simulink model "sf_elevator"  (R2017b)
settings: Solver=FixedStepDiscrete  StartTime=0.0  StopTime=inf  FixedStep=0.01  RelTol=1e-3  EnableMultiTasking=on
InitFcn:
  | allCarIds = [1 2];
StartFcn:
  | root = sfroot;
  | data = root.find('-isa','Stateflow.Data');
  | posA = data.find('Name','A_position').Props.InitialValue;
  | posB = data.find('Name','B_position').Props.InitialValue;
  | sf_elevator_gui('init', 'sf_elevator', allCarIds, [posA posB]);
StopFcn:
  | sf_elevator_gui('close');
undefined symbols (not defined in the file): Stateflow
libraries: sf_elevator_lib x2, sf_gui_elevator_controller_lib x2
CloseFcn:
  | sf_elevator_gui('close');
  | clear allCarIds;
settings Model: ExtModeAutoUpdateStatusClock=off  Creator=The MathWorks, Inc.  LastModifiedBy=The MathWorks, Inc.
settings DataIOCC: LimitDataPoints=on  SaveFormat=StructureWithTime  SignalLoggingName=sigsOut
settings OptimizationCC: ExpressionDepthLimit=2147483647  InitFltsAndDblsToZero=on  EfficientMapNaN2IntZero=off  LifeSpan=Inf
settings DebuggingCC: SaveWithParameterizedLinksMsg=none  UnderspecifiedInitializationDetection=Classic  MergeDetectMultiDrivingBlocksExec=none  SignalResolutionControl=TryResolveAllWithWarning  MultiTaskDSMMsg=warning  MultiTaskCondExecSysMsg=none  FcnCallInpInsideContextMsg=warning  AllowSymbolicDim=off  StateNameClashWarn=warning  SFUnexpectedBacktrackingDiag=warning  SFNoUnconditionalDefaultTransitionDiag=warning  SFExecutionAtInitializationDiag=none
settings HardwareCC: ProdBitPerPointer=32  ProdBitPerSizeT=32  ProdBitPerPtrDiffT=32  ProdLargestAtomicFloat=None  ProdIntDivRoundTo=Undefined  ProdEndianess=Unspecified  ProdWordSize=32  ProdHWDeviceType=32-bit Generic  TargetBitPerLong=64  TargetBitPerPointer=64  TargetBitPerSizeT=64  TargetBitPerPtrDiffT=64  TargetLongLongMode=on  TargetIntDivRoundTo=Zero  TargetEndianess=LittleEndian  TargetWordSize=64  TargetHWDeviceType=MATLAB Host  ProdEqTarget=off
settings ModelReferenceCC: PropagateSignalLabelsOutOfModel=off
settings SFSimCC: SFSimEcho=off  SimIntegrity=off  SimParseCustomCode=off
settings RTWCC: SystemTargetFile=ert.tlc  TemplateMakefile=ert_default_tmf  Description=Real-Time Workshop Embedded Coder  GenerateReport=on  IncludeHyperlinkInReport=on  LaunchReport=on  GenerateTraceInfo=on  GenerateTraceReport=on  GenerateTraceReportSl=on  GenerateTraceReportSf=on  GenerateTraceReportEml=on
settings CodeAppCC: IgnoreCustomStorageClasses=off  CustomSymbolStrType=$N$R$M  CustomSymbolStrModelFcn=$N  StateflowObjectComments=on  InternalIdentifier=Classic
settings ERTTargetCC: MultiwordLength=2048  GenerateSampleERTMain=on  ERTCustomFileTemplate=example_file_process.tlc  ConvertIfToSwitch=off  SuppressUnreachableDefaultCases=off
settings ConfigComp: CovMetricSettings=dcmtr  CovHtmlReporting=on  CovSaveCumulativeToWorkspaceVar=on  CovSaveSingleToWorkspaceVar=on  CovExternalEMLEnable=off  CovSFcnEnable=off

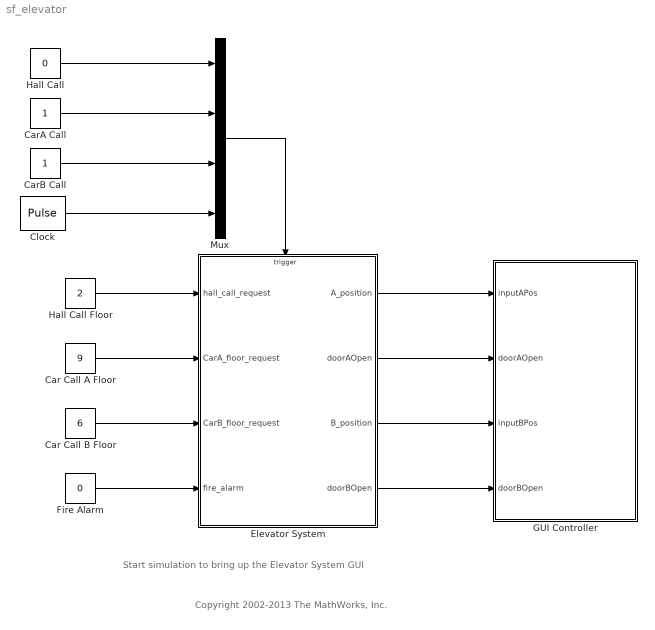
== system sf_elevator ==
  note: Start simulation to bring up the Elevator System GUI
  note: Copyright 2002-2013 The MathWorks, Inc.
  Car Call A Floor : Constant  Value=9  OutDataTypeStr=uint8
  Car Call B Floor : Constant  Value=6  OutDataTypeStr=uint8
  CarA Call : Constant  OutDataTypeStr=double
  CarB Call : Constant  OutDataTypeStr=double
  Clock : DiscretePulseGenerator  PulseType=Time based  PulseWidth=50
  Elevator System : Stateflow chart  TreatAsAtomicUnit=on
  Fire Alarm : Constant  Value=0  OutDataTypeStr=boolean
  GUI Controller : Stateflow chart  TreatAsAtomicUnit=on
  Hall Call : Constant  Value=0  OutDataTypeStr=double
  Hall Call Floor : Constant  Value=2  OutDataTypeStr=uint8
  Mux : Mux
  wires:
  Elevator System/1(A_position) -> GUI Controller/1(inputAPos)
  Elevator System/2(doorAOpen) -> GUI Controller/2(doorAOpen)
  Elevator System/3(B_position) -> GUI Controller/3(inputBPos)
  Elevator System/4(doorBOpen) -> GUI Controller/4(doorBOpen)
  Hall Call/1 -> Mux/1
  CarA Call/1 -> Mux/2
  CarB Call/1 -> Mux/3
  Clock/1 -> Mux/4
  Mux/1 -> Elevator System/Trigger
  Hall Call Floor/1 -> Elevator System/1(hall_call_request)
  Car Call A Floor/1 -> Elevator System/2(CarA_floor_request)
  Car Call B Floor/1 -> Elevator System/3(CarB_floor_request)
  Fire Alarm/1 -> Elevator System/4(fire_alarm)

== stateflow chart sf_elevator/Elevator System ==
  state Elevator_Manager [parallel]
    settings: executionOrder=1
    state register(hall_call_floor) [function]
      (default) -> (junction 2062) : {enqueue(hall_call_floor);
          | hall_call_status[hall_call_floor] = 1;}
    state enqueue(hall_call_floor) [function]
      (default) -> (junction 1513)
      (junction 1513) -> (junction 1514) [order 1] : [hall_call_status[hall_call_floor] != 0]
      (junction 1513) -> (junction 1516) [order 2] : {i = 0;}
      (junction 1516) -> (junction 1515) [order 1] : [hall_call_queue[i] == hall_call_floor]
      (junction 1516) -> (junction 1516) [order 2] : [hall_call_queue[i] > 0 && i<NUM_FLOOR]{i++;}
      (junction 1516) -> (junction 1517) [order 3]
      (junction 1517) -> (junction 1518) [order 1] : [i >= NUM_FLOOR]
      (junction 1517) -> (junction 1519) [order 2] : {hall_call_queue[i] = hall_call_floor;}
    state process_hall_call [function]
      (default) -> (junction 2070)
      (junction 2070) -> (junction 2072) : {
          | /* 'INIT':Initialization */
          | request_floor = hall_call_queue[0];
          | }
      (junction 2072) -> (junction 2074) : {
          | /* Fire alarm is on */
          | fire_alarm_on = (fire_alarm);
          | }
      (junction 2074) -> (junction 2076) : {
          | /* There is outstanding request */
          | request_outstanding = (request_floor > 0);
          | }
      (junction 2076) -> (junction 2078) : {
          | /* Elevator A is idle */
          | elevator_A_idle = (Elevator_A.get_status() == ElevatorStatus.IDLE);
          | }
      (junction 2078) -> (junction 2080) : {
          | /* Elevator B is idle */
          | elevator_B_idle = (Elevator_B.get_status() == ElevatorStatus.IDLE);
          | }
      (junction 2080) -> (junction 2082) : {
          | /* Elevator A is closer to request */
          | elevator_A_closer = (fabs(Elevator_A.get_position() - request_floor) <= fabs(Elevator_B.get_position() - request_floor));
          | }
      (junction 2082) -> (junction 2084) [order 1] : [fire_alarm_on]
      (junction 2084) -> (junction 2086) : {
          | /* 'EMR':Emergency */
          | Elevator_A.register(floor(Elevator_A.get_position()+Elevator_A.get_direction()/2));
          | Elevator_B.register(floor(Elevator_B.get_position()+Elevator_B.get_direction()/2));
          | }
      (junction 2082) -> (junction 2088) [order 2]
      (junction 2088) -> (junction 2090) [order 1] : [!request_outstanding]
      (junction 2090) -> (junction 2092) : {
          | /* 'NONE':Both elevators are busy, OR no request present */
          |
          | }
      (junction 2088) -> (junction 2094) [order 2]
      (junction 2094) -> (junction 2096) [order 1] : [!elevator_A_idle && !elevator_B_idle]
      (junction 2096) -> (junction 2098) : {
          | /* 'NONE':Both elevators are busy, OR no request present */
          |
          | }
      (junction 2094) -> (junction 2100) [order 2]
      (junction 2100) -> (junction 2102) [order 1] : [elevator_A_idle && !elevator_B_idle]
      (junction 2102) -> (junction 2104) : {
          | /* 'A':Elevator A should respond to request */
          | Elevator_A.enqueue(request_floor);
          | Main_dequeue(request_floor);
          | }
      (junction 2100) -> (junction 2106) [order 2]
      (junction 2106) -> (junction 2108) [order 1] : [!elevator_A_idle && elevator_B_idle]
      (junction 2108) -> (junction 2110) : {
          | /* 'B':Elevator B should respond to request */
          | Elevator_B.enqueue(request_floor);
          | Main_dequeue(request_floor);
          | }
      (junction 2106) -> (junction 2112) [order 2]
      (junction 2112) -> (junction 2114) [order 1] : [elevator_A_idle && elevator_B_idle && elevator_A_closer]
      (junction 2114) -> (junction 2116) : {
          | /* 'A':Elevator A should respond to request */
          | Elevator_A.enqueue(request_floor);
          | Main_dequeue(request_floor);
          | }
      (junction 2112) -> (junction 2118) [order 2]
      (junction 2118) -> (junction 2120) [order 1] : [elevator_A_idle && elevator_B_idle && !elevator_A_closer]
      (junction 2120) -> (junction 2122) : {
          | /* 'B':Elevator B should respond to request */
          | Elevator_B.enqueue(request_floor);
          | Main_dequeue(request_floor);
          | }
      (junction 2118) -> (junction 2124) [order 2]
    Elevator_Manager -> (junction 2054) [order 1] : HALL_CALL {register(hall_call_request);}
    Elevator_Manager -> (junction 2057) [order 2] : CLOCK {process_hall_call();} //Clock drives whole system
  state result = Main_exists_in_queue(floor) [function]
    (default) -> (junction 1904) : {i=0;}
    (junction 1904) -> (junction 1904) [order 1] : [hall_call_queue[i] > 0 && ...
        | i<NUM_FLOOR && ...
        | hall_call_queue[i] != floor]{i++;}
    (junction 1904) -> (junction 1905) [order 2]
    (junction 1905) -> (junction 1906) [order 1] : [i >= NUM_FLOOR || hall_call_queue[i] == 0]{result = 0;}
    (junction 1905) -> (junction 1907) [order 2] : {result = i+1;}
  state Main_deregister(hall_call_floor) [function]
    (default) -> (junction 1898) : {Main_dequeue(hall_call_floor);
        | hall_call_status[hall_call_floor] = 0;}
  state Elevator_A [parallel]
    settings: executionOrder=2
  state Main_dequeue(hall_call_floor) [function]
    (default) -> (junction 1916) : {i=0;}
    (junction 1916) -> (junction 1916) [order 1] : [hall_call_queue[i] > 0 && ...
        | i<NUM_FLOOR && ...
        | hall_call_queue[i] != hall_call_floor]{i++;}
    (junction 1916) -> (junction 1917) [order 2]
    (junction 1917) -> (junction 1918) [order 1] : [i >= NUM_FLOOR || hall_call_queue[i] == 0]
    (junction 1917) -> (junction 1919) [order 2]
    (junction 1919) -> (junction 1920) : {hall_call_queue[i] = hall_call_queue[i+1]; i++;}
    (junction 1920) -> (junction 1919) [order 1] : [i < NUM_FLOOR]
    (junction 1920) -> (junction 1921) [order 2]
  state Elevator_B [parallel]
    settings: executionOrder=3
  data: hall_call_floor function_input double; hall_call_floor function_input uint8; i temporary uint8; request_floor temporary uint8; fire_alarm_on temporary boolean =0; request_outstanding temporary boolean =0; elevator_A_idle temporary boolean =0; elevator_B_idle temporary boolean =0; elevator_A_closer temporary boolean =0; result function_output uint8; floor function_input uint8; i temporary uint8; hall_call_floor function_input uint8; i temporary uint8; hall_call_floor function_input uint8; hall_call_request input uint8; A_position output double =6; NUM_FLOOR constant uint8 =9; CarA_floor_request input uint8; CarB_floor_request input uint8; fire_alarm input boolean; hall_call_queue local uint8 size=10; hall_call_status local uint8 size=10; doorAOpen output boolean =0; B_position output double =1; doorBOpen output boolean =0
  data fire_alarm_on settings: description=Fire alarm is on
  data request_outstanding settings: description=There is outstanding request
  data elevator_A_idle settings: description=Elevator A is idle
  data elevator_B_idle settings: description=Elevator B is idle
  data elevator_A_closer settings: description=Elevator A is closer to request
  events: HALL_CALL input EITHER_EDGE_EVENT; CAR_CALL_A input EITHER_EDGE_EVENT; CAR_CALL_B input EITHER_EDGE_EVENT; CLOCK input EITHER_EDGE_EVENT

== stateflow chart sf_elevator/GUI Controller ==
  state CarA_Controller [parallel]
    settings: executionOrder=1
  state CarB_Controller [parallel]
    settings: executionOrder=2
  data: inputAPos input; doorAOpen input; inputBPos input; doorBOpen input; allCarIds parameter uint8 size=2
